simulink model "Simulator_tiltrotor"  (R2016b)
settings: Solver=ode45  StartTime=0.0  StopTime=simulation_time  RelTol=1e-3  EnableMultiTasking=on
InitFcn:
  | Parameters_physical_tiltrotor
undefined symbols (not defined in the file or in its folder): A_Servo, B_Servo, C_Servo, delay_attitude, delay_position, dLMN, gravity, inertia_rotor_hub, inertia_tensor, inertia_tensor_inv, Kq, Kt, mass, mass_matrix, mass_matrix_inv, motor_ome_vs_throttle, motor_tau, sample_time, sigbuilder_block
libraries: aerolibutil x10
(part 2 of 2)

== matlab function Simulator_tiltrotor/Tiltrotor/Actuators/dOmega_Pi and Omega_Pi computation 2/Time_derivative_rotation_matrix ==
  data: alpha_i input; dalpha_i input; dR_PiB output; motor_number input
function dR_PiB = Rot_matrix_dot(alpha_i, dalpha_i, motor_number)
%#codegen
phi = alpha_i;
psi = (motor_number - 1) * pi/2;

Sphi = sin(phi);
Cphi = cos(phi);
Spsi = sin(psi);
Cpsi = cos(psi);

Rx = [1   0     0  ;
      0 Cphi -Sphi ;
      0 Sphi  Cphi];
  
Rz = [Cpsi -Spsi 0 ;
      Spsi  Cpsi 0 ;
        0    0   1];
      
R_BPi = Rz * Rx;
R_PiB = R_BPi';

S = [ 0     0         0     ; 
      0     0     -dalpha_i ;
      0  dalpha_i     0    ];
 

dR_PiB = S * R_PiB;

== matlab function Simulator_tiltrotor/Tiltrotor/Actuators/External Momentum_3/O_BPi ==
  data: Origin_Pi output; motor_number input; arm_length parameter
 function Origin_Pi = Origin( motor_number, arm_length )
%#codegen
distance = [arm_length ;
                0      ;
                0     ];

psi = (motor_number - 1) * pi/2;

Spsi = sin(psi);
Cpsi = cos(psi);

Rz = [Cpsi -Spsi 0 ;
      Spsi  Cpsi 0 ;
        0    0   1];
      
Origin_Pi = Rz * distance;

== matlab function Simulator_tiltrotor/Tiltrotor/Actuators/External Momentum_3/Rotation_matrix ==
  data: R_BPi output; alpha_i input; motor_number input
function R_BPi = Rotation_matrix( alpha_i, motor_number )
%#codegen
% Rotation matrix from propeller group i-frame to body-frame
phi = alpha_i;
psi = (motor_number - 1) * pi/2;

Sphi = sin(phi);
Cphi = cos(phi);
Spsi = sin(psi);
Cpsi = cos(psi);

Rx = [1   0     0  ;
      0 Cphi -Sphi ;
      0 Sphi  Cphi];
  
Rz = [Cpsi -Spsi 0 ;
      Spsi  Cpsi 0 ;
        0    0   1];
      
R_BPi = Rz * Rx;

== matlab function Simulator_tiltrotor/Tiltrotor/Actuators/dOmega_Pi and Omega_Pi computation 1/Time_derivative_rotation_matrix ==
  data: alpha_i input; dalpha_i input; dR_PiB output; motor_number input
function dR_PiB = Rot_matrix_dot(alpha_i, dalpha_i, motor_number)
%#codegen
phi = alpha_i;
psi = (motor_number - 1) * pi/2;

Sphi = sin(phi);
Cphi = cos(phi);
Spsi = sin(psi);
Cpsi = cos(psi);

Rx = [1   0     0  ;
      0 Cphi -Sphi ;
      0 Sphi  Cphi];
  
Rz = [Cpsi -Spsi 0 ;
      Spsi  Cpsi 0 ;
        0    0   1];
      
R_BPi = Rz * Rx;
R_PiB = R_BPi';

S = [ 0     0         0     ; 
      0     0     -dalpha_i ;
      0  dalpha_i     0    ];
 

dR_PiB = S * R_PiB;

== matlab function Simulator_tiltrotor/Tiltrotor/Actuators/dOmega_Pi and Omega_Pi computation 3/Rotation_matrix ==
  data: R_PiB output; alpha_i input; motor_number input
function R_PiB = Rotation_matrix( alpha_i, motor_number )
%#codegen
% Rotation matrix from propeller group i-frame to body-frame
phi = alpha_i;
psi = (motor_number - 1) * pi/2;

Sphi = sin(phi);
Cphi = cos(phi);
Spsi = sin(psi);
Cpsi = cos(psi);

Rx = [1   0     0  ;
      0 Cphi -Sphi ;
      0 Sphi  Cphi];
  
Rz = [Cpsi -Spsi 0 ;
      Spsi  Cpsi 0 ;
        0    0   1];
      
R_BPi = Rz * Rx;
R_PiB = R_BPi';

== matlab function Simulator_tiltrotor/Tiltrotor/Actuators/dOmega_Pi and Omega_Pi computation 3/Time_derivative_rotation_matrix ==
  data: alpha_i input; dalpha_i input; dR_PiB output; motor_number input
function dR_PiB = Rot_matrix_dot(alpha_i, dalpha_i, motor_number)
%#codegen
phi = alpha_i;
psi = (motor_number - 1) * pi/2;

Sphi = sin(phi);
Cphi = cos(phi);
Spsi = sin(psi);
Cpsi = cos(psi);

Rx = [1   0     0  ;
      0 Cphi -Sphi ;
      0 Sphi  Cphi];
  
Rz = [Cpsi -Spsi 0 ;
      Spsi  Cpsi 0 ;
        0    0   1];
      
R_BPi = Rz * Rx;
R_PiB = R_BPi';

S = [ 0     0         0     ; 
      0     0     -dalpha_i ;
      0  dalpha_i     0    ];
 

dR_PiB = S * R_PiB;

== matlab function Simulator_tiltrotor/Tiltrotor/Actuators/Traslational Force_2/Rotation_matrix ==
  data: R_BPi output; alpha_i input; motor_number input
function R_BPi = Rotation_matrix( alpha_i, motor_number )
%#codegen
% Rotation matrix from propeller group i-frame to body-frame
phi = alpha_i;
psi = (motor_number - 1) * pi/2;

Sphi = sin(phi);
Cphi = cos(phi);
Spsi = sin(psi);
Cpsi = cos(psi);

Rx = [1   0     0  ;
      0 Cphi -Sphi ;
      0 Sphi  Cphi];
  
Rz = [Cpsi -Spsi 0 ;
      Spsi  Cpsi 0 ;
        0    0   1];
      
R_BPi = Rz * Rx;

== matlab function Simulator_tiltrotor/Tiltrotor/Actuators/Traslational Force_3/Rotation_matrix ==
  data: R_BPi output; alpha_i input; motor_number input
function R_BPi = Rotation_matrix( alpha_i, motor_number )
%#codegen
% Rotation matrix from propeller group i-frame to body-frame
phi = alpha_i;
psi = (motor_number - 1) * pi/2;

Sphi = sin(phi);
Cphi = cos(phi);
Spsi = sin(psi);
Cpsi = cos(psi);

Rx = [1   0     0  ;
      0 Cphi -Sphi ;
      0 Sphi  Cphi];
  
Rz = [Cpsi -Spsi 0 ;
      Spsi  Cpsi 0 ;
        0    0   1];
      
R_BPi = Rz * Rx;

== matlab function Simulator_tiltrotor/Tiltrotor/Actuators/Traslational Force_4/Rotation_matrix ==
  data: R_BPi output; alpha_i input; motor_number input
function R_BPi = Rotation_matrix( alpha_i, motor_number )
%#codegen
% Rotation matrix from propeller group i-frame to body-frame
phi = alpha_i;
psi = (motor_number - 1) * pi/2;

Sphi = sin(phi);
Cphi = cos(phi);
Spsi = sin(psi);
Cpsi = cos(psi);

Rx = [1   0     0  ;
      0 Cphi -Sphi ;
      0 Sphi  Cphi];
  
Rz = [Cpsi -Spsi 0 ;
      Spsi  Cpsi 0 ;
        0    0   1];
      
R_BPi = Rz * Rx;

== matlab function Simulator_tiltrotor/Tiltrotor/Actuators/External Momentum_4/O_BPi ==
  data: Origin_Pi output; motor_number input; arm_length parameter
 function Origin_Pi = Origin( motor_number, arm_length )
%#codegen
distance = [arm_length ;
                0      ;
                0     ];

psi = (motor_number - 1) * pi/2;

Spsi = sin(psi);
Cpsi = cos(psi);

Rz = [Cpsi -Spsi 0 ;
      Spsi  Cpsi 0 ;
        0    0   1];
      
Origin_Pi = Rz * distance;

== matlab function Simulator_tiltrotor/Tiltrotor/Actuators/External Momentum_1/O_BPi ==
  data: Origin_Pi output; motor_number input; arm_length parameter
 function Origin_Pi = Origin( motor_number, arm_length )
%#codegen
distance = [arm_length ;
                0      ;
                0     ];

psi = (motor_number - 1) * pi/2;

Spsi = sin(psi);
Cpsi = cos(psi);

Rz = [Cpsi -Spsi 0 ;
      Spsi  Cpsi 0 ;
        0    0   1];
      
Origin_Pi = Rz * distance;

== matlab function Simulator_tiltrotor/Tiltrotor/Actuators/External Momentum_4/Rotation_matrix ==
  data: R_BPi output; alpha_i input; motor_number input
function R_BPi = Rotation_matrix( alpha_i, motor_number )
%#codegen
% Rotation matrix from propeller group i-frame to body-frame
phi = alpha_i;
psi = (motor_number - 1) * pi/2;

Sphi = sin(phi);
Cphi = cos(phi);
Spsi = sin(psi);
Cpsi = cos(psi);

Rx = [1   0     0  ;
      0 Cphi -Sphi ;
      0 Sphi  Cphi];
  
Rz = [Cpsi -Spsi 0 ;
      Spsi  Cpsi 0 ;
        0    0   1];
      
R_BPi = Rz * Rx;

== matlab function Simulator_tiltrotor/Tiltrotor/Actuators/dOmega_Pi and Omega_Pi computation 1/Rotation_matrix ==
  data: R_PiB output; alpha_i input; motor_number input
function R_PiB = Rotation_matrix( alpha_i, motor_number )
%#codegen
% Rotation matrix from propeller group i-frame to body-frame
phi = alpha_i;
psi = (motor_number - 1) * pi/2;

Sphi = sin(phi);
Cphi = cos(phi);
Spsi = sin(psi);
Cpsi = cos(psi);

Rx = [1   0     0  ;
      0 Cphi -Sphi ;
      0 Sphi  Cphi];
  
Rz = [Cpsi -Spsi 0 ;
      Spsi  Cpsi 0 ;
        0    0   1];
      
R_BPi = Rz * Rx;
R_PiB = R_BPi';

== matlab function Simulator_tiltrotor/Tiltrotor/Actuators/dOmega_Pi and Omega_Pi computation 4/Rotation_matrix ==
  data: R_PiB output; alpha_i input; motor_number input
function R_PiB = Rotation_matrix( alpha_i, motor_number )
%#codegen
% Rotation matrix from propeller group i-frame to body-frame
phi = alpha_i;
psi = (motor_number - 1) * pi/2;

Sphi = sin(phi);
Cphi = cos(phi);
Spsi = sin(psi);
Cpsi = cos(psi);

Rx = [1   0     0  ;
      0 Cphi -Sphi ;
      0 Sphi  Cphi];
  
Rz = [Cpsi -Spsi 0 ;
      Spsi  Cpsi 0 ;
        0    0   1];
      
R_BPi = Rz * Rx;
R_PiB = R_BPi';

== matlab function Simulator_tiltrotor/Tiltrotor/Actuators/dOmega_Pi and Omega_Pi computation 4/Time_derivative_rotation_matrix ==
  data: alpha_i input; dalpha_i input; dR_PiB output; motor_number input
function dR_PiB = Rot_matrix_dot(alpha_i, dalpha_i, motor_number)
%#codegen
phi = alpha_i;
psi = (motor_number - 1) * pi/2;

Sphi = sin(phi);
Cphi = cos(phi);
Spsi = sin(psi);
Cpsi = cos(psi);

Rx = [1   0     0  ;
      0 Cphi -Sphi ;
      0 Sphi  Cphi];
  
Rz = [Cpsi -Spsi 0 ;
      Spsi  Cpsi 0 ;
        0    0   1];
      
R_BPi = Rz * Rx;
R_PiB = R_BPi';

S = [ 0     0         0     ; 
      0     0     -dalpha_i ;
      0  dalpha_i     0    ];
 

dR_PiB = S * R_PiB;

== matlab function Simulator_tiltrotor/Tiltrotor/Actuators/External Momentum_1/Rotation_matrix ==
  data: R_BPi output; alpha_i input; motor_number input
function R_BPi = Rotation_matrix( alpha_i, motor_number )
%#codegen
% Rotation matrix from propeller group i-frame to body-frame
phi = alpha_i;
psi = (motor_number - 1) * pi/2;

Sphi = sin(phi);
Cphi = cos(phi);
Spsi = sin(psi);
Cpsi = cos(psi);

Rx = [1   0     0  ;
      0 Cphi -Sphi ;
      0 Sphi  Cphi];
  
Rz = [Cpsi -Spsi 0 ;
      Spsi  Cpsi 0 ;
        0    0   1];
      
R_BPi = Rz * Rx;
